simulink model "HW_7_2_2C"  (R2019b)
settings: Solver=VariableStepAuto  StartTime=0.0  StopTime=50  RelTol=1e-3  EnableMultiTasking=on
settings Model: Creator=Teng-Hu  LastModifiedBy=liu
settings DataIOCC: ReturnWorkspaceOutputs=off
settings OptimizationCC: LifeSpan=inf
settings DebuggingCC: SFUnexpectedBacktrackingDiag=warning  SFNoUnconditionalDefaultTransitionDiag=warning  SFExecutionAtInitializationDiag=none  ArithmeticOperatorsInVariantConditions=warning
settings SFSimCC: SimUseLocalCustomCode=off  CustomCodeUndefinedFunction=UseInterfaceOnly
settings RTWCC: RTWUseLocalCustomCode=off
settings CodeAppCC: StateflowObjectComments=on
settings GRTTargetCC: TargetLangStandard=C89/C90 (ANSI)
settings ConfigComp: CovMetricSettings=dw  CovHtmlReporting=on  CovSaveCumulativeToWorkspaceVar=on  CovSaveSingleToWorkspaceVar=on  CovExternalEMLEnable=off

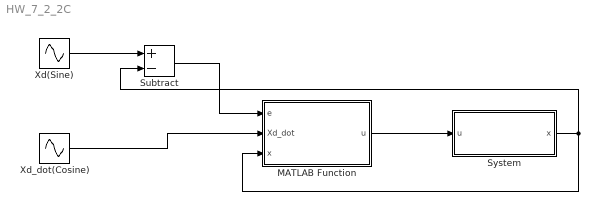
== system HW_7_2_2C ==
  MATLAB Function : MATLAB Function  TreatAsAtomicUnit=on
  Subtract : Sum  Inputs=+-
  System : Subsystem
  Xd(Sine) : Sin  SampleTime=0
  Xd_dot(Cosine) : Sin  Phase=pi/2  SampleTime=0
  wires:
  MATLAB Function/1(u) -> System/1(u)
  Xd_dot(Cosine)/1 -> MATLAB Function/2(Xd_dot)
  System/1(x) -> MATLAB Function/3(x), Subtract/2
  Xd(Sine)/1 -> Subtract/1
  Subtract/1 -> MATLAB Function/1(e)

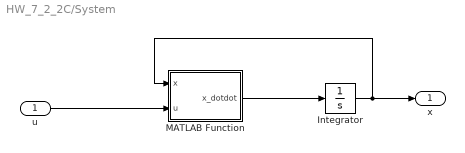
== system HW_7_2_2C/System ==
  u : Inport
  Integrator : Integrator  InitialCondition=1
  MATLAB Function : MATLAB Function  TreatAsAtomicUnit=on
  x : Outport
  wires:
  Integrator/1 -> MATLAB Function/1(x), x/1
  u/1 -> MATLAB Function/2(u)
  MATLAB Function/1(x_dotdot) -> Integrator/1

== matlab function HW_7_2_2C/MATLAB Function ==
  data: e input; Xd_dot input; u output; x input
function u = fcn(e, Xd_dot, x)
a = 2;
b = 5;
k = 10;
u = Xd_dot + k*e - a*x - b*cos(x);

== matlab function HW_7_2_2C/System/MATLAB Function ==
  data: x input; u input; x_dotdot output
function x_dotdot = fcn(x,u)
%#codegen

x_dotdot = 2*x+5*cos(x)+u;
